simulink model "FlameAnalysis"  (R2015b)
settings: Solver=ode45  SolverMode=SingleTasking  StartTime=0.0  StopTime=1000  RelTol=1e-3
PreLoadFcn:
  | fprintf('loading now...\n')
PostLoadFcn:
  | model_name = gcs;
  | video_player_name=[model_name, '/From Multimedia File'];
  | video_path=get_param(video_player_name,'inputFileName');
  | model_path= get_param(model_name,'filename');
  | i=findstr('\',model_path);
  | 
  | if(~exist(video_path))
  |      video_path2=[model_path(1:i(end))  video_path(findstr('Video',video_path):end)];
  | 
  |      if(exist(video_path2))
  |           set_param(video_player_name,'inputFileName',video_path2);
  |      else
  |           j=findstr('\',video_path);
  |           video_path2=[model_path(1:i(end))  'Videos\' video_path(j(end)+1:end)];
  |           if(exist(video_path2))
  |                set_param(video_player_name,'inputFileName',video_path2);
  |           else
  |                avifiles=dir('videos\*.avi')
  |                set_param(video_player_name,'inputFileName',[model_path(1:i(end))  'Videos\'   avifiles(1).name]);
  |           end
  | 
  |      end
  | end
InitFcn:
  | clc
  | clear
  | global  t position wide dz_dt d2z_dt2 d3z_dt3 Af As dA_dt filePath Su_ Su alfa Karlovitz threshold model_name bords tWalls sheet model_path simulating numPointsAnalysis
  | simulating=true;
  | model_name = gcs;
  | model_path = [model_name, '/Edit Parameters'];
  | tbf = str2num(get_param(model_path,'tbf'));
  | ppcm= str2num(get_param(model_path,'ppcm'));
  | p2e= str2num(get_param(model_path,'p2e'));
  | 
  | nframes0= str2num(get_param(model_path,'nframes0'));
  | alfa= str2num(get_param(model_path,'alfa'));
  | fff= str2num(get_param(model_path,'fff'));
  | 
  | if((size(fff,2)~=1) & (size(fff,2)~=2))
  |     error('The flame front fraction must be scalar or 1x2-array');
  | end
  | order=str2num(get_param(model_path,'order'));
  | numberOfPoints=str2num(get_param(model_path,'numberOfPoints'));
  | orderAnalysis=str2num(get_param(model_path,'orderAnalysis'));
  | numPointsAnalysis=str2num(get_param(model_path,'numPointsAnalysis'));
  | uselog=str2num(get_param(model_path,'uselog'));
  | 
  | 
  | save2xls= strcmp('on',get_param(model_path,'save2xls'));
  | saveVideo= strcmp('on',get_param(model_path,'saveVideo'));
  | cfs= strcmp('on',get_param(model_path,'cfs'));
  | c3dv= strcmp('on',get_param(model_path,'c3dv'));
  | 
  | 
  | if(strcmp(get_param(model_path,'bge'),'Temporal Median Estimator'))
  |      bge=1;
  | elseif (strcmp(get_param(model_path,'bge'),'Temporal Median'))
  |     bge=2;
  |     bkgnd{1}=[gcs '/Background Estimator/Decomposing Red Movement/BG1/Temporal Median/Temporal Median'];
  |     bkgnd{2}=[gcs '/Background Estimator/Decomposing Green Movement/BG1/Temporal Median/Temporal Median'];
  |     bkgnd{3}=[gcs '/Background Estimator/Decomposing Blue Movement/BG1/Temporal Median/Temporal Median'];
  | 
  |     nframes0=max(nframes0,1);
  |     set_param([gcs '/Edit Parameters/'],'nframes0',num2str(nframes0));
  |     for i=1:3
  |         set_param(bkgnd{i}, 'tw', num2str(nframes0));
  |     end
  | else
  |     bge=3;
  | end
  | 
  | 
  | 
  | switch(get_param(model_path,'aprox_type'))
  |      case 'Profile'
  |            aprox_type=1;
  |            sheet='Profile';
  |      case 'Paraboloid (moving base)'
  |            aprox_type=2;
  |            sheet='Paraboloid';
  |      case 'Paraboloid(fixed base)'
  |            aprox_type=3;
  |            sheet='ParaboloidFB';
  |      case 'Spheroid'
  |            aprox_type=4;
  |            sheet='Spheroid';
  |      case 'Profile Spheroid'
  |            aprox_type=5;
  |            sheet='Profile Spheroid';
  | end
  | 
  | 
  | video_player_name=[model_name, '/From Multimedia File'];
  | video_path=get_param(video_player_name,'inputFileName');
  | video_name=getVideoNameFromPath(video_path);
  | hVideoSrc = vision.VideoFileReader(video_path, ...
  |                    'ImageColorSpace','Intensity');
  | firstFrame=step(hVideoSrc);
  | clear hVideoSrc;
  | [m n]=size(firstFrame);
  | 
  | 
  | set_param([model_name '/Display Results/Save Video/modified video/'],'outputFilename',['Videos Matlab/' video_name '_' get_param(model_path,'aprox_type') '_Matlab.avi']);
StopFcn:
  | global editing  simulating
  | simulating = true;
  | try
  |       closeFunction
  | catch err
  |       simulating=false;
  |       err
  | end
  |   simulating=false;
model workspace (MATLAB code in the model file):
  | line_row =  22;
values from neighbouring files (symbols this model uses):
  m = size(BW,1)    [flameFront.m]    (also in putCircles.m = (y(i+1)-y(i))./(x(i+1)-x(i)))
  n = n(n==size(num,2)/4)    [averageOfVideos.m]    (also in countFramesOfVideo.m = 1; putCircles.m = length(y))
  vector = cast([row, col],'double')    [flameFront.m]
undefined symbols (not defined in the file or in its folder): strel
libraries: simulink x27, visionstatistics x14, visionconversions x9, visiontextngfix x9, visionmorphops x7, dspvision x4, visionsinks x2, visiongeotforms x1
(part 1 of 3)
CloseFcn:
  | fprintf('closing now...\n')
settings Model: NumberOfSteps=10  ExtModeAutoUpdateStatusClock=off  Creator=don  LastModifiedBy=nicku
settings DataIOCC: SaveFormat=Array
settings OptimizationCC: BlockReduction=off  BooleanDataType=off
settings DebuggingCC: SaveWithParameterizedLinksMsg=none  UnderspecifiedInitializationDetection=Classic  MergeDetectMultiDrivingBlocksExec=none
settings HardwareCC: ProdBitPerPointer=32  ProdLargestAtomicFloat=None  ProdIntDivRoundTo=Undefined  ProdEndianess=Unspecified  ProdWordSize=32  ProdHWDeviceType=32-bit Generic  TargetUnknown=on
settings GRTTargetCC: GeneratePreprocessorConditionals=Disable all
settings ConfigComp: CovModelRefEnable=Off  CovSFcnEnable=off

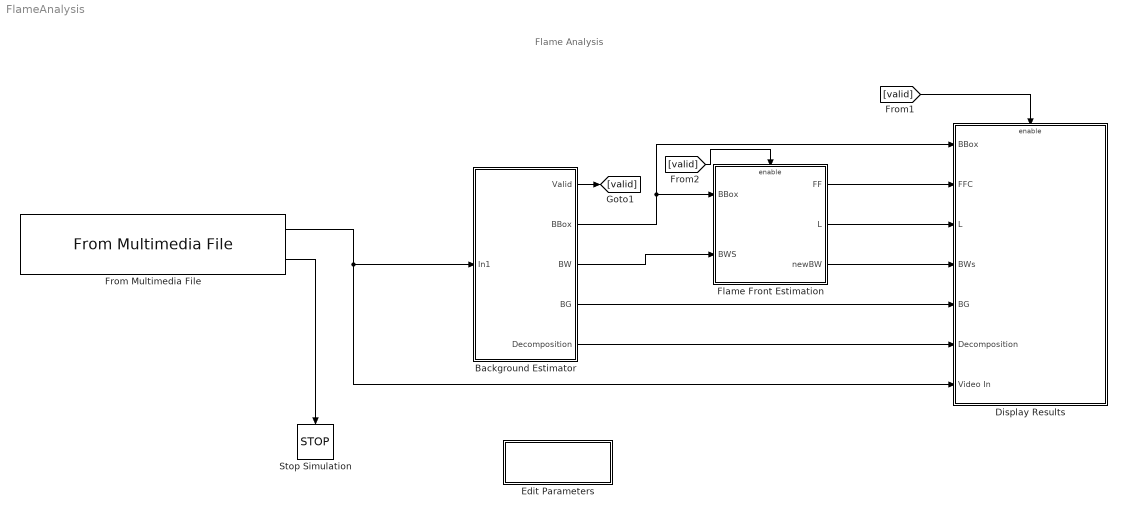
== system FlameAnalysis ==
  note: Flame Analysis
  Background Estimator : Subsystem
  Display Results : Subsystem
  Edit Parameters : Subsystem  mask(Edit Parameters){saveVideo=on, save2xls=on, cfs=on, c3dv=off, bge=Temporal Median, nframes0=52, fff=[0.95        0.93], tbf=200, ppcm=(781 -84)/85, p2e=88, alfa=951.18/293.15, numberOfPoints=10, order=3, aprox_type=Profile Spheroid, splinesmoothing=Spline Smoothing (matlab), numPointsAnalysis=[0.95        0.98       0.001], orderAnalysis=[3  3], uselog=[2  2  1]}
      mask prompts: saveVideo "Save Video"; save2xls "Save Data to excel"; cfs "Calculate Flame Surface"; c3dv "Create 3D video"; bge "Background Estimator"; nframes0 "Number of initial frames"; fff "Flame Front Fraction (0-1)"; tbf "Time Between Frames (microsecs)"; ppcm "Pixels per centimeter (cm^ -1)"; p2e "Number of pixels between the bottom and the electrodes"; numberOfPoints "Number of Points for regression of Flame Profile"; order "Order Of  polynomial regresion of flame profile"; aprox_type "Type of aproximation for flame front"; splinesmoothing "Method for ploynomial regression"; numPointsAnalysis "Smoothing Parameter"; orderAnalysis "Order of polynomia for data regresion  for area and position derivatives"; uselog "Use regression logaritms"
      mask init:
      | % global editing smoothing
      | % model_path=[gcs '/Edit Parameters'];
      | % smoothing=strcmp(get_param(model_path,'splinesmoothing'),'Spline Smoothing (matlab)');
      | % if ~editing
      | %     
      | % 
      | % a=getSimulinkBlockHandle(model_path,true);
      | % masknames=get(a, 'masknames'); 
      | % maskprompts=get(a, 'maskprompts');
      | % maskvisibilities=get(a, 'maskvisibilities');
      | % 
      | % inp=cellfun(@(x)strcmp(x,'numPointsAnalysis'),masknames);
      | % ioa=cellfun(@(x)strcmp(x,'orderAnalysis'),masknames);
      | % 
      | % 
      | % if strcmp(get_param(model_path,'splinesmoothing'),'Spline Smoothing (matlab)')
      | %     maskprompts{inp}='Smoothing Parameter';
      | %     maskvisibilities{ioa}='off';
      | %     set_param(model_path,'numPointsAnalysis',['[' num2str(10.^(log10(str2num(get_param(model_path,'numPointsAnalysis')))+4)) ']']);
      | % else
      | %     maskprompts{inp}='Number of Points for regression of Flame Profile';
      | %     maskvisibilities{ioa}='on';
      | %     set_param(model_path,'numPointsAnalysis',['[' num2str(round(10.^(log10(str2num(get_param(model_path,'numPointsAnalysis')))-4))) ']']);
      | % end
      | % 
      | % set(a,'maskprompts',maskprompts);
      | % set(a,'maskvisibilities',maskvisibilities);
      | % 
      | % end
      settings: RTWMemSecFuncInitTerm=Default  RTWMemSecFuncExecute=Default  RTWMemSecDataConstants=Default  RTWMemSecDataInternal=Default  RTWMemSecDataParameters=Default
      mask TypeOptions bge: Temporal Median Estimator | Temporal Median | Motion Based Background Estimator
      mask TypeOptions aprox_type: Profile | Paraboloid (moving base) | Paraboloid(fixed base) | Spheroid | Profile Spheroid
      mask TypeOptions splinesmoothing: Spline Smoothing (matlab) | multipolyfit  (nicolas' sad try to do what matlab already does)
      mask Callback splinesmoothing:
      | % global editing smoothing
      | % model_path=[gcs '/Edit Parameters'];
      | % if ~editing & strcmp(get_param(model_path,'splinesmoothing'),'Spline Smoothing (matlab)')~=smoothing
      | %     model_path=[gcs '/Edit Parameters'];
      | %
      | % a=getSimulinkBlockHandle(model_path,true);
      | % masknames=get(a, 'masknames');
      | % maskprompts=get(a, 'maskprompts');
      | % maskvisibilities=get(a, 'maskvisibilities');
      | %
      | % inp=cellfun(@(x)strcmp(x,'numPointsAnalysis'),masknames);
      | % ioa=cellfun(@(x)strcmp(x,'orderAnalysis'),masknames);
      | %
      | %
      | % if strcmp(get_param(model_path,'splinesmoothing'),'Spline Smoothing (matlab)')
      | %     maskprompts{inp}='Smoothing Parameter';
      | %     maskvisibilities{ioa}='off';
      | %     set_param(model_path,'numPointsAnalysis',['[' num2str(10.^(log10(str2num(get_param(model_path,'numPointsAnalysis')))-4)) ']']);
      | % else
      | %     maskprompts{inp}='Number of Points for regression of Flame Profile';
      | %     maskvisibilities{ioa}='on';
      | %     set_param(model_path,'numPointsAnalysis',['[' num2str(round(10.^(log10(str2num(get_param(model_path,'numPointsAnalysis')))+4))) ']']);
      | % end
      | %
      | % set(a,'maskprompts',maskprompts);
      | % set(a,'maskvisibilities',maskvisibilities);
      | %
      | % end
      | % smoothing= strcmp(get_param(model_path,'splinesmoothing'),'Spline Smoothing (matlab)');
      mask Display: disp('Edit\nParameters')
  Flame Front Estimation : Subsystem
  From Multimedia File : dspvision/From Multimedia File  inputFilename=D:\Documents\LRGP\GitHub\Flame Detection\Videos\Amidon_319mg_Methane_8.47%_tv120ms_1000mJ_2VD.avi  loop=on  numPlays=2  outputStreams=Video only  videoDataType=single  audioDataType=int16  inheritSampleTime=on  userDefinedSampleTime=1/40  noAudioOutput=off  isIntensityVideo=off  fourcc=RGB  colorVideoFormat=One multidimensional signal  outputEOF=on  dataOrg=Column-major  audioFrameSize=1024  computeAudioFrameSize=off  outSamplingMode=Frame based
  Stop Simulation : Stop
  wires:
  [valid] -> Flame Front Estimation/Enable
  Flame Front Estimation/1(FF) -> Display Results/2(FFC)
  From Multimedia File/2 -> Stop Simulation/1
  Flame Front Estimation/2(L) -> Display Results/3(L)
  [valid] -> Display Results/Enable
  Flame Front Estimation/3(newBW) -> Display Results/4(BWs)
  Background Estimator/2(BBox) -> Display Results/1(BBox), Flame Front Estimation/1(BBox)
  Background Estimator/1(Valid) -> [valid]
  Background Estimator/3(BW) -> Flame Front Estimation/2(BWS)
  Background Estimator/4(BG) -> Display Results/5(BG)
  From Multimedia File/1 -> Display Results/7(Video In), Background Estimator/1(In1)
  Background Estimator/5(Decomposition) -> Display Results/6(Decomposition)

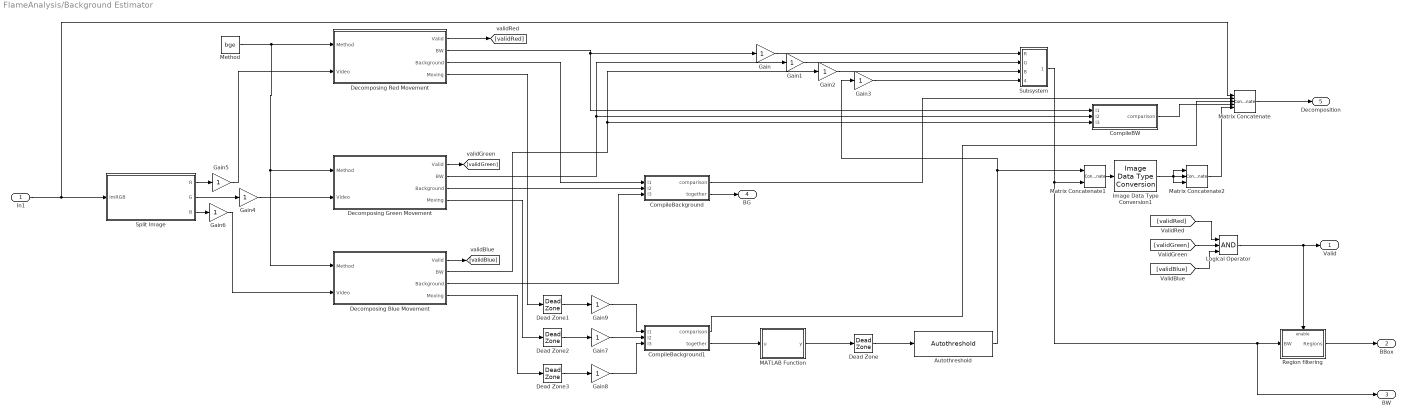
== system FlameAnalysis/Background Estimator ==
  In1 : Inport
  Autothreshold : visionconversions/Autothreshold  operator=>  threshOut=off  effMetricOut=off  userDefinedRange=off  umin=0  umax=255  outOfRngOpt=Warn and saturate  scaleThreshold=off  scaleFactor=0.011  P1Mode=Specify word length  P1WordLength=32  P1FracLength=30  P2Mode=Specify word length  P2WordLength=32  P2FracLength=22  P3Mode=Specify word length  P3WordLength=32  P3FracLength=14  P4Mode=Binary point scaling  P4WordLength=32  P4FracLength=15  Q1Mode=Specify word length  Q1WordLength=32  Q1FracLength=16  EMMode=Specify word length  EMWordLength=16  EMFracLength=14  roundingMode=Floor  overflowMode=off
  CompileBW : MATLAB Function  TreatAsAtomicUnit=on
  CompileBackground : MATLAB Function  TreatAsAtomicUnit=on
  CompileBackground1 : MATLAB Function  TreatAsAtomicUnit=on
  Dead Zone{,1..3} (4 alike) : DeadZone  LowerValue=0  UpperValue=0  SaturateOnIntegerOverflow=on
  Decomposing Blue Movement : Subsystem
  Decomposing Green Movement : Subsystem
  Decomposing Red Movement : Subsystem
  Gain{,1..9} (10 alike) : Gain
  Image Data Type Conversion1 : visionconversions/Image Data Type Conversion  outDT=single  isSigned=on  wordLen=16  numFracBits=0
  Logical Operator : Logic  Inputs=3  AllPortsSameDT=off  OutDataTypeStr=boolean
  MATLAB Function : MATLAB Function  TreatAsAtomicUnit=on
  Matrix Concatenate : Concatenate  NumInputs=5  Mode=Multidimensional array
  Matrix Concatenate1 : Concatenate  Mode=Multidimensional array
  Matrix Concatenate2 : Concatenate  NumInputs=3  Mode=Multidimensional array  ConcatenateDimension=3
  Method : Constant  Value=bge  OutDataTypeStr=single
  Region filtering : Subsystem
      settings: RTWMemSecFuncInitTerm=Default  RTWMemSecFuncExecute=Default  RTWMemSecDataConstants=Default  RTWMemSecDataInternal=Default  RTWMemSecDataParameters=Default
  Split Image : MATLAB Function  TreatAsAtomicUnit=on
  Subsystem : Subsystem
  Valid : Outport
  BBox : Outport  Port=2
  BW : Outport  Port=3
  BG : Outport  Port=4
  Decomposition : Outport  Port=5
  wires:
  Logical Operator/1 -> Valid/1, Region filtering/Enable
  Region filtering/1(Regions) -> BBox/1
  Subsystem/1(BW) -> Matrix Concatenate1/2, BW/1, Region filtering/1(BW)
  CompileBackground/2(together) -> BG/1
  Method/1 -> Decomposing Blue Movement/1(Method), Decomposing Green Movement/1(Method), Decomposing Red Movement/1(Method)
  Decomposing Red Movement/2(BW) -> CompileBW/1(I1), Gain/1
  Decomposing Red Movement/3(Background) -> CompileBackground/1(I1)
  Decomposing Red Movement/1(Valid) -> [validRed]
  Decomposing Green Movement/1(Valid) -> [validGreen]
  Decomposing Blue Movement/1(Valid) -> [validBlue]
  [validRed] -> Logical Operator/1
  [validGreen] -> Logical Operator/2
  [validBlue] -> Logical Operator/3
  Decomposing Green Movement/3(Background) -> CompileBackground/2(I2)
  Decomposing Blue Movement/3(Background) -> CompileBackground/3(I3)
  Decomposing Green Movement/2(BW) -> Gain1/1, CompileBW/2(I2)
  Decomposing Blue Movement/2(BW) -> Gain2/1, CompileBW/3(I3)
  Matrix Concatenate/1 -> Decomposition/1
  CompileBackground1/2(together) -> MATLAB Function/1(u)
  CompileBackground/1(comparison) -> Matrix Concatenate/2
  CompileBackground1/1(comparison) -> Matrix Concatenate/3
  CompileBW/1(comparison) -> Matrix Concatenate/4
  Matrix Concatenate2/1 -> Matrix Concatenate/5
  Gain/1 -> Subsystem/1(R)
  Gain1/1 -> Subsystem/2(G)
  Gain2/1 -> Subsystem/3(B)
  Gain3/1 -> Subsystem/4(RGB)
  Autothreshold/1 -> Gain3/1, Matrix Concatenate1/1
  Matrix Concatenate1/1 -> Image Data Type Conversion1/1
  Image Data Type Conversion1/1 -> Matrix Concatenate2/1, Matrix Concatenate2/3, Matrix Concatenate2/2
  Split Image/1(R) -> Gain5/1
  Split Image/2(G) -> Gain4/1
  Split Image/3(B) -> Gain6/1
  Decomposing Green Movement/4(Moving) -> Dead Zone2/1
  Decomposing Blue Movement/4(Moving) -> Dead Zone3/1
  Decomposing Red Movement/4(Moving) -> Dead Zone1/1
  In1/1 -> Matrix Concatenate/1, Split Image/1(imRGB)
  Gain4/1 -> Decomposing Green Movement/2(Video)
  Gain5/1 -> Decomposing Red Movement/2(Video)
  Gain6/1 -> Decomposing Blue Movement/2(Video)
  Dead Zone/1 -> Autothreshold/1
  MATLAB Function/1(y) -> Dead Zone/1
  Dead Zone1/1 -> Gain9/1
  Dead Zone2/1 -> Gain7/1
  Dead Zone3/1 -> Gain8/1
  Gain7/1 -> CompileBackground1/2(I2)
  Gain8/1 -> CompileBackground1/3(I3)
  Gain9/1 -> CompileBackground1/1(I1)

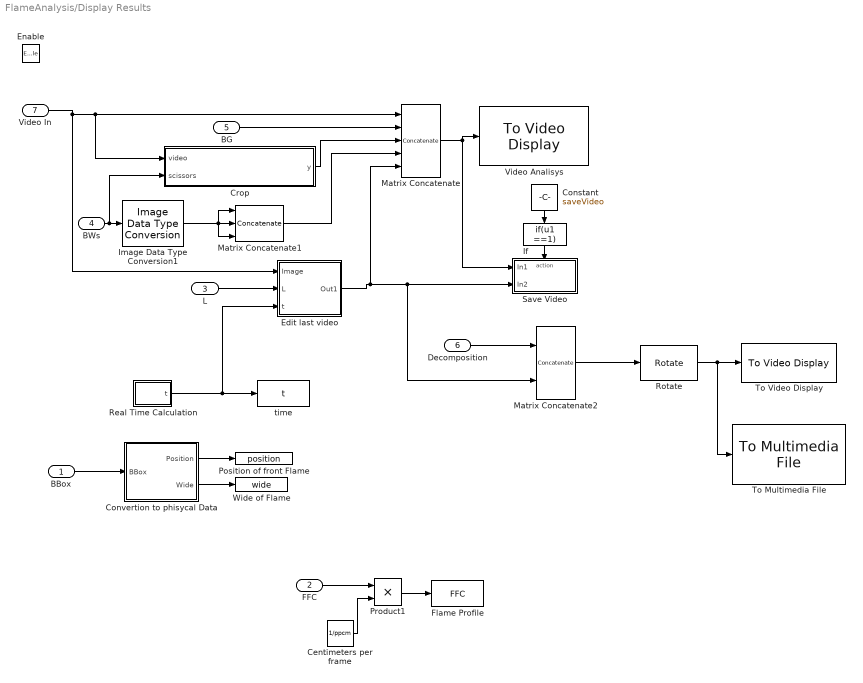
== system FlameAnalysis/Display Results ==
  BBox : Inport
  FFC : Inport  Port=2
  L : Inport  Port=3
  BWs : Inport  Port=4
  BG : Inport  Port=5
  Decomposition : Inport  Port=6
  Video In : Inport  Port=7
  Enable : EnablePort  PropagateVarSize=During execution
  Centimeters per frame : Constant  Value=1/ppcm
  Constant : Constant  Value=saveVideo
  Convertion to phisycal Data : Subsystem
  Crop : MATLAB Function  TreatAsAtomicUnit=on
  Edit last video : Subsystem
  Flame Profile : ToWorkspace  VariableName=FFC  SaveFormat=Structure With Time  SampleTime=-1
  If : If  IfExpression=u1 ==1  ShowElse=off
  Image Data Type Conversion1 : visionconversions/Image Data Type Conversion  outDT=single  isSigned=on  wordLen=16  numFracBits=0
  Matrix Concatenate : Concatenate  NumInputs=5  Mode=Multidimensional array
  Matrix Concatenate1 : Concatenate  NumInputs=3  Mode=Multidimensional array  ConcatenateDimension=3
  Matrix Concatenate2 : Concatenate  Mode=Multidimensional array
  Position of front Flame : ToWorkspace  VariableName=position  SampleTime=-1
  Product1 : Product  RndMeth=Zero
  Real Time Calculation : Subsystem
  Rotate : visiongeotforms/Rotate  outSizeR=Expanded to fit rotated input image  src_angle=Specify via dialog  unit_angle=Degrees  angle=pi/2  maxAngle=pi  dispImage=Center  method=Table lookup  fillVal=0  interpMethod=Bilinear  prodOutputMode=Binary point scaling  prodOutputWordLength=32  prodOutputFracLength=10  roundingMode=Nearest  overflowMode=on
  Save Video : Subsystem  TreatAsAtomicUnit=on
  To Multimedia File : dspvision/To Multimedia File  outputFilename=Videos Matlab\decomposition.avi  streamSelection=Video only  videoCompressor=None (uncompressed)  audioCompressor=None (uncompressed)  imagePorts=One multidimensional signal  fileType=AVI  audioDatatype=Determine from input data type  fourcc=RGB  videoQuality=75  mj2000CompFactor=10
  To Video Display : visionsinks/To Video Display  windowSizeMode=True size (1:1)  openAtMdlStart=on  fullScreen=off  videoWindowX=-1920  videoWindowY=-104  saveWindowSize=off  videoWindowWidth=1920  videoWindowHeight=1017  inputColorFormat=RGB  inputType=Obsolete  imagePorts=One multidimensional signal  OutputDevice=On-screen video monitor  dataOrg=Column-major  isWindowOpen=on
  Video Analisys : visionsinks/To Video Display  windowSizeMode=True size (1:1)  openAtMdlStart=on  fullScreen=off  videoWindowX=0  videoWindowY=23  saveWindowSize=off  videoWindowWidth=1366  videoWindowHeight=705  inputColorFormat=RGB  inputType=Obsolete  imagePorts=One multidimensional signal  OutputDevice=On-screen video monitor  dataOrg=Column-major  isWindowOpen=on
  Wide of Flame : ToWorkspace  VariableName=wide  SampleTime=-1
  time : ToWorkspace  VariableName=t  SampleTime=-1
  wires:
  BWs/1 -> Crop/2(scissors), Image Data Type Conversion1/1
  Matrix Concatenate/1 -> Save Video/1(In1), Video Analisys/1
  Video In/1 -> Edit last video/1(Image), Crop/1(video), Matrix Concatenate/1
  BBox/1 -> Convertion to phisycal Data/1(BBox)
  Convertion to phisycal Data/1(Position) -> Position of front Flame/1
  Convertion to phisycal Data/2(Wide) -> Wide of Flame/1
  Constant/1 -> If/1
  If/1 -> Save Video/Action
  Real Time Calculation/1(t) -> time/1, Edit last video/3(t)
  FFC/1 -> Product1/1
  Centimeters per frame/1 -> Product1/2
  Product1/1 -> Flame Profile/1
  Edit last video/1(Out1) -> Matrix Concatenate/5, Matrix Concatenate2/2, Save Video/2(In2)
  L/1 -> Edit last video/2(L)
  Image Data Type Conversion1/1 -> Matrix Concatenate1/1, Matrix Concatenate1/3, Matrix Concatenate1/2
  BG/1 -> Matrix Concatenate/2
  Matrix Concatenate1/1 -> Matrix Concatenate/4
  Crop/1(y) -> Matrix Concatenate/3
  Decomposition/1 -> Matrix Concatenate2/1
  Rotate/1 -> To Multimedia File/1, To Video Display/1
  Matrix Concatenate2/1 -> Rotate/1

== system FlameAnalysis/Edit Parameters ==

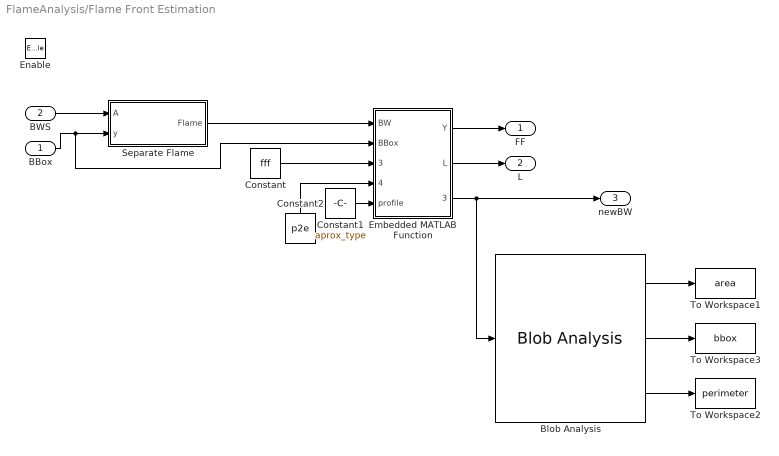
== system FlameAnalysis/Flame Front Estimation ==
  BBox : Inport
  BWS : Inport  Port=2
  Enable : EnablePort  PropagateVarSize=During execution
  Blob Analysis : visionstatistics/Blob Analysis  Tag=vipblks_row_conv  area=on  centroid=off  bBox=on  majorAxis=off  minorAxis=off  angle=off  eccentricity=off  equivDiameterSq=off  extent=off  perimeter=on  maxBlobs=1  warnIfNumBlobsExceeded=on  isCount=off  useMinArea=off  minArea=5*5  useMaxArea=off  maxArea=intmax('uint32')  excludeBorderBlob=off  outDT=double  isOutVarDim=off  isFill=on  fillValues=-1  conn=8  isLabel=off  outputMode=Binary point scaling  outputWordLength=32  outputFracLength=16  firstCoeffMode=Binary point scaling  firstCoeffWordLength=16  firstCoeffFracLength=14  secondCoeffMode=Binary point scaling  secondCoeffWordLength=32  secondCoeffFracLength=16  accumMode=Binary point scaling  accumWordLength=32  accumFracLength=0  prodOutputMode=Binary point scaling  prodOutputWordLength=32  prodOutputFracLength=16  roundingMode=Floor  overflowMode=off
  Constant : Constant  Value=fff  VectorParams1D=off
  Constant1 : Constant  Value=aprox_type  VectorParams1D=off
  Constant2 : Constant  Value=p2e  VectorParams1D=off
  Embedded MATLAB Function : MATLAB Function  TreatAsAtomicUnit=on
  Separate Flame : MATLAB Function  TreatAsAtomicUnit=on
  To Workspace1 : ToWorkspace  VariableName=area  SampleTime=-1
  To Workspace2 : ToWorkspace  VariableName=perimeter  SampleTime=-1
  To Workspace3 : ToWorkspace  VariableName=bbox  SampleTime=-1
  FF : Outport
  L : Outport  Port=2
  newBW : Outport  Port=3
  wires:
  BWS/1 -> Separate Flame/1(A)
  BBox/1 -> Separate Flame/2(y), Embedded MATLAB Function/2(BBox)
  Separate Flame/1(Flame) -> Embedded MATLAB Function/1(BW)
  Constant/1 -> Embedded MATLAB Function/3(fraction)
  Constant1/1 -> Embedded MATLAB Function/5(profile)
  Embedded MATLAB Function/1(Y) -> FF/1
  Embedded MATLAB Function/2(L) -> L/1
  Constant2/1 -> Embedded MATLAB Function/4(y_electrodes)
  Embedded MATLAB Function/3(newBW) -> Blob Analysis/1, newBW/1
  Blob Analysis/1 -> To Workspace1/1
  Blob Analysis/3 -> To Workspace2/1
  Blob Analysis/2 -> To Workspace3/1

== system FlameAnalysis/Background Estimator/Decomposing Blue Movement ==
  Method : Inport
  Video : Inport  Port=2
  BG1 : Subsystem
  Movement Tracker : Subsystem
  Valid : Outport
  BW : Outport  Port=2
  Background : Outport  Port=3
  Moving : Outport  Port=4
  wires:
  Video/1 -> BG1/2(Video), Movement Tracker/2(Video In 1)
  Method/1 -> BG1/1(Constant)
  BG1/2(Background) -> Background/1, Movement Tracker/1(Background 1)
  Movement Tracker/2(BW) -> BW/1
  BG1/1(Valid) -> Movement Tracker/Enable, Valid/1
  Movement Tracker/1(Moving) -> Moving/1

== system FlameAnalysis/Background Estimator/Decomposing Green Movement ==
  Method : Inport
  Video : Inport  Port=2
  BG1 : Subsystem
  Movement Tracker : Subsystem
  Valid : Outport
  BW : Outport  Port=2
  Background : Outport  Port=3
  Moving : Outport  Port=4
  wires:
  Video/1 -> BG1/2(Video), Movement Tracker/2(Video In 1)
  Movement Tracker/1(Moving) -> Moving/1
  Method/1 -> BG1/1(Constant)
  BG1/2(Background) -> Background/1, Movement Tracker/1(Background 1)
  Movement Tracker/2(BW) -> BW/1
  BG1/1(Valid) -> Movement Tracker/Enable, Valid/1

== system FlameAnalysis/Background Estimator/Decomposing Red Movement ==
  Method : Inport
  Video : Inport  Port=2
  BG1 : Subsystem
  Movement Tracker : Subsystem
  Valid : Outport
  BW : Outport  Port=2
  Background : Outport  Port=3
  Moving : Outport  Port=4
  wires:
  Video/1 -> BG1/2(Video), Movement Tracker/2(Video In 1)
  Movement Tracker/1(Moving) -> Moving/1
  Method/1 -> BG1/1(Constant)
  BG1/2(Background) -> Background/1, Movement Tracker/1(Background 1)
  Movement Tracker/2(BW) -> BW/1
  BG1/1(Valid) -> Movement Tracker/Enable, Valid/1

== system FlameAnalysis/Background Estimator/Region filtering ==
  BW : Inport
  Enable : EnablePort  PropagateVarSize=During execution
  Blob Analysis : visionstatistics/Blob Analysis  Tag=vipblks_row_conv  area=on  centroid=off  bBox=on  majorAxis=off  minorAxis=off  angle=off  eccentricity=off  equivDiameterSq=off  extent=off  perimeter=off  maxBlobs=1000  warnIfNumBlobsExceeded=on  isCount=off  useMinArea=off  minArea=5*5  useMaxArea=on  maxArea=int32(0.9*m*n)  excludeBorderBlob=off  outDT=double  isOutVarDim=off  isFill=on  fillValues=0  conn=8  isLabel=off  outputMode=Binary point scaling  outputWordLength=32  outputFracLength=16  firstCoeffMode=Binary point scaling  firstCoeffWordLength=16  firstCoeffFracLength=14  secondCoeffMode=Binary point scaling  secondCoeffWordLength=32  secondCoeffFracLength=16  accumMode=Binary point scaling  accumWordLength=32  accumFracLength=0  prodOutputMode=Binary point scaling  prodOutputWordLength=32  prodOutputFracLength=16  roundingMode=Floor  overflowMode=off
  blobDepurator : MATLAB Function  TreatAsAtomicUnit=on
  Regions : Outport
  wires:
  BW/1 -> Blob Analysis/1
  Blob Analysis/2 -> blobDepurator/2(blobs)
  Blob Analysis/1 -> blobDepurator/1(areas)
  blobDepurator/1(Y) -> Regions/1

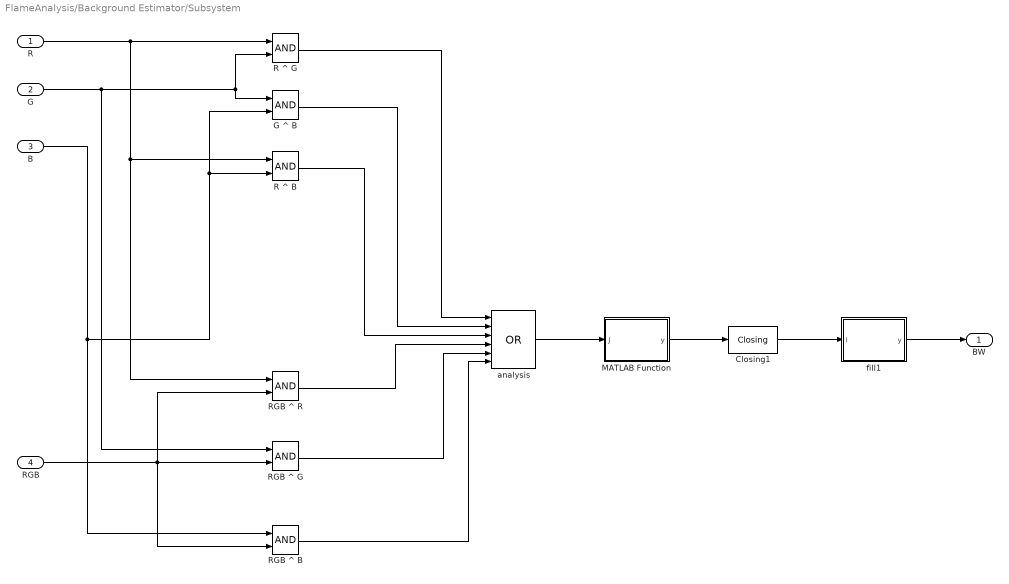
== system FlameAnalysis/Background Estimator/Subsystem ==
  R : Inport
  G : Inport  Port=2
  B : Inport  Port=3
  RGB : Inport  Port=4
  Closing1 : visionmorphops/Closing  nhoodsrc=Specify via dialog  strel=strel('disk',3)
  G ^ B : Logic  AllPortsSameDT=off  OutDataTypeStr=boolean
  MATLAB Function : MATLAB Function  TreatAsAtomicUnit=on
  R ^ B : Logic  AllPortsSameDT=off  OutDataTypeStr=boolean
  R ^ G : Logic  AllPortsSameDT=off  OutDataTypeStr=boolean
  RGB ^ B : Logic  AllPortsSameDT=off  OutDataTypeStr=boolean
  RGB ^ G : Logic  AllPortsSameDT=off  OutDataTypeStr=boolean
  RGB ^ R : Logic  AllPortsSameDT=off  OutDataTypeStr=boolean
  analysis : Logic  Operator=OR  Inputs=6  AllPortsSameDT=off  OutDataTypeStr=boolean
  fill1 : MATLAB Function  TreatAsAtomicUnit=on
  BW : Outport
  wires:
  R/1 -> RGB ^ R/1, R ^ B/1, R ^ G/1
  G/1 -> RGB ^ G/1, G ^ B/1, R ^ G/2
  B/1 -> RGB ^ B/1, R ^ B/2, G ^ B/2
  R ^ G/1 -> analysis/1
  G ^ B/1 -> analysis/2
  R ^ B/1 -> analysis/3
  analysis/1 -> MATLAB Function/1(J)
  RGB/1 -> RGB ^ B/2, RGB ^ G/2, RGB ^ R/2
  RGB ^ R/1 -> analysis/4
  RGB ^ G/1 -> analysis/5
  RGB ^ B/1 -> analysis/6
  MATLAB Function/1(y) -> Closing1/1
  fill1/1(y) -> BW/1
  Closing1/1 -> fill1/1(I)

== system FlameAnalysis/Display Results/Convertion to phisycal Data ==
  BBox : Inport
  Array To Scalar : MATLAB Function  TreatAsAtomicUnit=on
  Centimeters per frame : Constant  Value=1/ppcm
  pixels to electrodes : Constant  Value=p2e
  Position : Outport
  Wide : Outport  Port=2
  wires:
  Array To Scalar/1(position) -> Position/1
  BBox/1 -> Array To Scalar/1(u)
  pixels to electrodes/1 -> Array To Scalar/3(p2e)
  Centimeters per frame/1 -> Array To Scalar/2(cmpf)
  Array To Scalar/2(wide) -> Wide/1

== system FlameAnalysis/Display Results/Edit last video ==
  Image : Inport
  L : Inport  Port=2
  t : Inport  Port=3
  Constant : Constant  Value=int32([n/2-35 m-20 80 30])
  Draw Shapes : visiontextngfix/Draw Shapes  shape=Rectangles  fill=on  lineWidth=1  fillClrSource=Specify via dialog  display=Black  intensity=200  color=[255 0 0]  opacity=1  viewport=Entire image  antialiasing=off  inType=Obsolete  imagePorts=One multidimensional signal  prodOutputMode=Binary point scaling  prodOutputWordLength=32  prodOutputFracLength=14  memoryMode=Specify word length  memoryWordLength=16  memoryFracLength=14  roundingMode=Floor  overflowMode=off
  Draw Shapes1 : visiontextngfix/Draw Shapes  shape=Lines  fill=off  lineWidth=1  fillClrSource=Specify via dialog  display=User-specified value  intensity=200  color=[ 0 0 0]  opacity=0.6  viewport=Entire image  antialiasing=off  inType=Obsolete  imagePorts=One multidimensional signal  prodOutputMode=Binary point scaling  prodOutputWordLength=32  prodOutputFracLength=14  memoryMode=Specify word length  memoryWordLength=16  memoryFracLength=14  roundingMode=Floor  overflowMode=off
  Insert Text : visiontextngfix/Insert Text  inputType=Obsolete  theText=['%6.2f ms']  getTextLocFrom=Specify via dialog  textLoc=int32([n/2-30 m-15])  getTextColorFrom=Specify via dialog  textColor=[1 1 1]  getTextIntensityFrom=Specify via dialog  textIntensity=0  getTextOpacityFrom=Specify via dialog  textOpacity=1.0  dummyVar2=0  dummyVar3=0  dummyVar4=0  imagePorts=One multidimensional signal  isInputTransposed=off  fontFace=LucidaSansRegular  dummyVar1=0  blockFontSize=12  antiAliased=on
  Out1 : Outport
  wires:
  Image/1 -> Draw Shapes1/1
  L/1 -> Draw Shapes1/2
  t/1 -> Insert Text/2
  Insert Text/1 -> Out1/1
  Draw Shapes/1 -> Insert Text/1
  Draw Shapes1/1 -> Draw Shapes/1
  Constant/1 -> Draw Shapes/2

== system FlameAnalysis/Display Results/Real Time Calculation ==
  Constant : Constant  Value=tbf/1000
  Constant1 : Constant
  Frame Counter : Subsystem
  Product : Product  RndMeth=Zero
  Sum : Sum  Inputs=|-+
  t : Outport
  wires:
  Frame Counter/1(" Cnt") -> Sum/2
  Constant/1 -> Product/2
  Constant1/1 -> Sum/1
  Sum/1 -> Product/1
  Product/1 -> t/1

== system FlameAnalysis/Display Results/Save Video ==
  In1 : Inport
  In2 : Inport  Port=2
  Action Port : ActionPort  ActionType=then
  Whole video : dspvision/To Multimedia File  outputFilename=Videos Matlab\results2.avi  streamSelection=Video only  videoCompressor=None (uncompressed)  audioCompressor=None (uncompressed)  imagePorts=One multidimensional signal  fileType=AVI  audioDatatype=Determine from input data type  fourcc=RGB  videoQuality=75  mj2000CompFactor=10
  modified video : dspvision/To Multimedia File  outputFilename=Videos Matlab/Amidon_319mg_Methane_8.47%_tv120ms_1000mJ_2VD_Profile Spheroid_Matlab.avi  streamSelection=Video only  videoCompressor=None (uncompressed)  audioCompressor=None (uncompressed)  imagePorts=One multidimensional signal  fileType=AVI  audioDatatype=Determine from input data type  fourcc=RGB  videoQuality=75  mj2000CompFactor=10
  wires:
  In1/1 -> Whole video/1
  In2/1 -> modified video/1

== system FlameAnalysis/Background Estimator/Decomposing Blue Movement/BG1 ==
  Constant : Inport
  Video : Inport  Port=2
  Compare To Constant : simulink/Logic and Bit Operations/Compare To Constant  relop===  const=1  OutDataTypeStr=boolean  ZeroCross=off
  Compare To Constant1 : simulink/Logic and Bit Operations/Compare To Constant  relop===  const=2  OutDataTypeStr=boolean  ZeroCross=off
  Compare To Constant2 : simulink/Logic and Bit Operations/Compare To Constant  relop===  const=3  OutDataTypeStr=boolean  ZeroCross=off
  Merge : Merge  Inputs=3
  Merge1 : Merge  Inputs=3
  Motion Based Background Estimator : Subsystem
  Temporal Median : Subsystem
  Temporal Median Estimator : Subsystem
  Valid : Outport
  Background : Outport  Port=2
  wires:
  Video/1 -> Motion Based Background Estimator/1(In), Temporal Median/1(In), Temporal Median Estimator/1(In)
  Constant/1 -> Compare To Constant1/1, Compare To Constant2/1, Compare To Constant/1
  Merge1/1 -> Valid/1
  Compare To Constant2/1 -> Motion Based Background Estimator/Enable
  Motion Based Background Estimator/1(BG) -> Merge/3
  Temporal Median Estimator/1(BG) -> Merge/1
  Merge/1 -> Background/1
  Compare To Constant1/1 -> Temporal Median/Enable
  Temporal Median/1(BG) -> Merge/2
  Temporal Median Estimator/2(Valid) -> Merge1/1
  Temporal Median/2(Valid) -> Merge1/2
  Motion Based Background Estimator/2(Valid) -> Merge1/3
  Compare To Constant/1 -> Temporal Median Estimator/Enable

== system FlameAnalysis/Background Estimator/Decomposing Blue Movement/Movement Tracker ==
  Background 1 : Inport
  Video In 1 : Inport  Port=2
  Enable : EnablePort  PropagateVarSize=During execution
  Abs3 : Abs  SaturateOnIntegerOverflow=on
  Autothreshold : visionconversions/Autothreshold  operator=>  threshOut=off  effMetricOut=off  userDefinedRange=off  umin=0  umax=255  outOfRngOpt=Warn and saturate  scaleThreshold=off  scaleFactor=0.011  P1Mode=Specify word length  P1WordLength=32  P1FracLength=30  P2Mode=Specify word length  P2WordLength=32  P2FracLength=22  P3Mode=Specify word length  P3WordLength=32  P3FracLength=14  P4Mode=Binary point scaling  P4WordLength=32  P4FracLength=15  Q1Mode=Specify word length  Q1WordLength=32  Q1FracLength=16  EMMode=Specify word length  EMWordLength=16  EMFracLength=14  roundingMode=Floor  overflowMode=off
  Dead Zone : DeadZone  LowerValue=0  UpperValue=0.05  SaturateOnIntegerOverflow=on
  Gain : Gain
  Sum1 : Sum  Inputs=-+  SaturateOnIntegerOverflow=on  InputSameDT=on  OutDataTypeStr=Inherit: Same as first input
  Moving : Outport
  BW : Outport  Port=2
  wires:
  Video In 1/1 -> Sum1/2
  Sum1/1 -> Abs3/1
  Background 1/1 -> Sum1/1
  Autothreshold/1 -> BW/1
  Dead Zone/1 -> Gain/1
  Abs3/1 -> Dead Zone/1
  Gain/1 -> Moving/1, Autothreshold/1

== system FlameAnalysis/Background Estimator/Decomposing Green Movement/BG1 ==
  Constant : Inport
  Video : Inport  Port=2
  Compare To Constant : simulink/Logic and Bit Operations/Compare To Constant  relop===  const=1  OutDataTypeStr=boolean  ZeroCross=off
  Compare To Constant1 : simulink/Logic and Bit Operations/Compare To Constant  relop===  const=2  OutDataTypeStr=boolean  ZeroCross=off
  Compare To Constant2 : simulink/Logic and Bit Operations/Compare To Constant  relop===  const=3  OutDataTypeStr=boolean  ZeroCross=off
  Merge : Merge  Inputs=3
  Merge1 : Merge  Inputs=3
  Motion Based Background Estimator : Subsystem
  Temporal Median : Subsystem
  Temporal Median Estimator : Subsystem
  Valid : Outport
  Background : Outport  Port=2
  wires:
  Video/1 -> Motion Based Background Estimator/1(In), Temporal Median/1(In), Temporal Median Estimator/1(In)
  Constant/1 -> Compare To Constant1/1, Compare To Constant2/1, Compare To Constant/1
  Merge1/1 -> Valid/1
  Compare To Constant2/1 -> Motion Based Background Estimator/Enable
  Motion Based Background Estimator/1(BG) -> Merge/3
  Temporal Median Estimator/1(BG) -> Merge/1
  Merge/1 -> Background/1
  Compare To Constant1/1 -> Temporal Median/Enable
  Temporal Median/1(BG) -> Merge/2
  Temporal Median Estimator/2(Valid) -> Merge1/1
  Temporal Median/2(Valid) -> Merge1/2
  Motion Based Background Estimator/2(Valid) -> Merge1/3
  Compare To Constant/1 -> Temporal Median Estimator/Enable

== system FlameAnalysis/Background Estimator/Decomposing Green Movement/Movement Tracker ==
  Background 1 : Inport
  Video In 1 : Inport  Port=2
  Enable : EnablePort  PropagateVarSize=During execution
  Abs3 : Abs  SaturateOnIntegerOverflow=on
  Autothreshold : visionconversions/Autothreshold  operator=>  threshOut=off  effMetricOut=off  userDefinedRange=off  umin=0  umax=255  outOfRngOpt=Warn and saturate  scaleThreshold=off  scaleFactor=2  P1Mode=Specify word length  P1WordLength=32  P1FracLength=30  P2Mode=Specify word length  P2WordLength=32  P2FracLength=22  P3Mode=Specify word length  P3WordLength=32  P3FracLength=14  P4Mode=Binary point scaling  P4WordLength=32  P4FracLength=15  Q1Mode=Specify word length  Q1WordLength=32  Q1FracLength=16  EMMode=Specify word length  EMWordLength=16  EMFracLength=14  roundingMode=Floor  overflowMode=off
  Dead Zone : DeadZone  LowerValue=0  UpperValue=0  SaturateOnIntegerOverflow=on
  Gain : Gain
  Sum1 : Sum  Inputs=-+  SaturateOnIntegerOverflow=on  InputSameDT=on  OutDataTypeStr=Inherit: Same as first input
  Moving : Outport
  BW : Outport  Port=2
  wires:
  Video In 1/1 -> Sum1/2
  Sum1/1 -> Abs3/1
  Background 1/1 -> Sum1/1
  Abs3/1 -> Dead Zone/1
  Autothreshold/1 -> BW/1
  Dead Zone/1 -> Gain/1
  Gain/1 -> Autothreshold/1, Moving/1

== system FlameAnalysis/Background Estimator/Decomposing Red Movement/BG1 ==
  Constant : Inport
  Video : Inport  Port=2
  Compare To Constant : simulink/Logic and Bit Operations/Compare To Constant  relop===  const=1  OutDataTypeStr=boolean  ZeroCross=off
  Compare To Constant1 : simulink/Logic and Bit Operations/Compare To Constant  relop===  const=2  OutDataTypeStr=boolean  ZeroCross=off
  Compare To Constant2 : simulink/Logic and Bit Operations/Compare To Constant  relop===  const=3  OutDataTypeStr=boolean  ZeroCross=off
  Merge : Merge  Inputs=3
  Merge1 : Merge  Inputs=3
  Motion Based Background Estimator : Subsystem
  Temporal Median : Subsystem
  Temporal Median Estimator : Subsystem
  Valid : Outport
  Background : Outport  Port=2
  wires:
  Video/1 -> Motion Based Background Estimator/1(In), Temporal Median/1(In), Temporal Median Estimator/1(In)
  Constant/1 -> Compare To Constant1/1, Compare To Constant2/1, Compare To Constant/1
  Merge1/1 -> Valid/1
  Compare To Constant2/1 -> Motion Based Background Estimator/Enable
  Motion Based Background Estimator/1(BG) -> Merge/3
  Temporal Median Estimator/1(BG) -> Merge/1
  Merge/1 -> Background/1
  Compare To Constant1/1 -> Temporal Median/Enable
  Temporal Median/1(BG) -> Merge/2
  Temporal Median Estimator/2(Valid) -> Merge1/1
  Temporal Median/2(Valid) -> Merge1/2
  Motion Based Background Estimator/2(Valid) -> Merge1/3
  Compare To Constant/1 -> Temporal Median Estimator/Enable

== system FlameAnalysis/Background Estimator/Decomposing Red Movement/Movement Tracker ==
  Background 1 : Inport
  Video In 1 : Inport  Port=2
  Enable : EnablePort  PropagateVarSize=During execution
  Abs3 : Abs  SaturateOnIntegerOverflow=on
  Autothreshold : visionconversions/Autothreshold  operator=>  threshOut=off  effMetricOut=off  userDefinedRange=off  umin=0  umax=255  outOfRngOpt=Warn and saturate  scaleThreshold=off  scaleFactor=5  P1Mode=Specify word length  P1WordLength=32  P1FracLength=30  P2Mode=Specify word length  P2WordLength=32  P2FracLength=22  P3Mode=Specify word length  P3WordLength=32  P3FracLength=14  P4Mode=Binary point scaling  P4WordLength=32  P4FracLength=15  Q1Mode=Specify word length  Q1WordLength=32  Q1FracLength=16  EMMode=Specify word length  EMWordLength=16  EMFracLength=14  roundingMode=Floor  overflowMode=off
  Dead Zone : DeadZone  LowerValue=0  UpperValue=0.2  SaturateOnIntegerOverflow=on
  Sum1 : Sum  Inputs=-+  SaturateOnIntegerOverflow=on  InputSameDT=on  OutDataTypeStr=Inherit: Same as first input
  Moving : Outport
  BW : Outport  Port=2
  wires:
  Video In 1/1 -> Sum1/2
  Sum1/1 -> Abs3/1
  Background 1/1 -> Sum1/1
  Autothreshold/1 -> BW/1
  Abs3/1 -> Dead Zone/1
  Dead Zone/1 -> Autothreshold/1, Moving/1

== system FlameAnalysis/Display Results/Real Time Calculation/Frame Counter ==
  Constant : Constant  OutDataTypeStr=int32
  Delay : Delay  DelayLength=1  InitialCondition=0  InputProcessing=Inherited
  Sum : Sum  Inputs=++|  OutDataTypeStr=Inherit: Same as first input
  " Cnt" : Outport
  wires:
  Delay/1 -> Sum/1
  Sum/1 -> " Cnt"/1, Delay/1
  Constant/1 -> Sum/2

== system FlameAnalysis/Background Estimator/Decomposing Blue Movement/BG1/Motion Based Background Estimator ==
  In : Inport
  Enable : EnablePort  PropagateVarSize=During execution
  Motion Based Background Estimator : Subsystem  mask(Motion Based Background Estimation){}
      mask help: The block uses the first few frames of the video stream to estimate the background image. It subtracts the background from each video frame to produce foreground images and only redraws the portion of the background that is revealed by the moving objects.
      mask Display: disp('Motion Based\nBackground\nEstimator')
  Signal Conversion : SignalConversion  ConversionOutput=Contiguous copy
  Signal Conversion1 : SignalConversion  ConversionOutput=Contiguous copy
  BG : Outport
  Valid : Outport  Port=2  InitialOutput=0
  wires:
  Signal Conversion1/1 -> Valid/1
  Signal Conversion/1 -> BG/1
  Motion Based Background Estimator/2(Valid) -> Signal Conversion1/1
  Motion Based Background Estimator/1(BG) -> Signal Conversion/1
  In/1 -> Motion Based Background Estimator/1(In)

== system FlameAnalysis/Background Estimator/Decomposing Blue Movement/BG1/Temporal Median ==
  In : Inport
  Enable : EnablePort  PropagateVarSize=During execution
  Temporal Median : Subsystem  mask(Temporal Median){tw=52}
      mask prompts: tw "Enter the number of frames over which to compute the median:"
      mask help: Computes median values of a series of video frames.
      mask Display: disp('Temporal\nMedian')
  BG : Outport
  Valid : Outport  Port=2  InitialOutput=0
  wires:
  In/1 -> Temporal Median/1(In)
  Temporal Median/1(BG) -> BG/1
  Temporal Median/2(Valid) -> Valid/1

== system FlameAnalysis/Background Estimator/Decomposing Blue Movement/BG1/Temporal Median Estimator ==
  In : Inport
  Enable : EnablePort  PropagateVarSize=During execution
  Signal Conversion : SignalConversion  ConversionOutput=Contiguous copy
  Temporal Median Estimator : Subsystem  mask(Temporal Median Estimator){t0=2}
      mask prompts: t0 "Number of frames after which the median is valid:"
      mask help: This block estimates the median values of the video data over time. The accuracy of the estimate improves with each new video frame.
      mask Help:
      | The running median estimation algorithm updates the past median of time series data based upon the knowledge of the new data sample. The past median is incremented or decremented based on how the new sample compares to the old median by an amount determined by standard error of the estimate. A special correction is also applied when a local ramp is detected in the time series data attempting to push the estimate to follow the same ramp trend.
      | 
      | The estimated median is then constrained within Chebychev's bounds which are sqrt(3/5) of standard deviation either side of the mean of the data.
      mask Display: disp('Temporal\nMedian\nEstimator')
  BG : Outport
  Valid : Outport  Port=2  InitialOutput=0
  wires:
  Signal Conversion/1 -> BG/1
  Temporal Median Estimator/2(Valid) -> Valid/1
  Temporal Median Estimator/1(BG) -> Signal Conversion/1
  In/1 -> Temporal Median Estimator/1(In)

== system FlameAnalysis/Background Estimator/Decomposing Green Movement/BG1/Motion Based Background Estimator ==
  In : Inport
  Enable : EnablePort  PropagateVarSize=During execution
  Motion Based Background Estimator : Subsystem  mask(Motion Based Background Estimation){}
      mask help: The block uses the first few frames of the video stream to estimate the background image. It subtracts the background from each video frame to produce foreground images and only redraws the portion of the background that is revealed by the moving objects.
      mask Display: disp('Motion Based\nBackground\nEstimator')
  Signal Conversion : SignalConversion  ConversionOutput=Contiguous copy
  Signal Conversion1 : SignalConversion  ConversionOutput=Contiguous copy
  BG : Outport
  Valid : Outport  Port=2  InitialOutput=0
  wires:
  Signal Conversion1/1 -> Valid/1
  Signal Conversion/1 -> BG/1
  Motion Based Background Estimator/2(Valid) -> Signal Conversion1/1
  Motion Based Background Estimator/1(BG) -> Signal Conversion/1
  In/1 -> Motion Based Background Estimator/1(In)

== system FlameAnalysis/Background Estimator/Decomposing Green Movement/BG1/Temporal Median ==
  In : Inport
  Enable : EnablePort  PropagateVarSize=During execution
  Temporal Median : Subsystem  mask(Temporal Median){tw=52}
      mask prompts: tw "Enter the number of frames over which to compute the median:"
      mask help: Computes median values of a series of video frames.
      mask Display: disp('Temporal\nMedian')
  BG : Outport
  Valid : Outport  Port=2  InitialOutput=0
  wires:
  In/1 -> Temporal Median/1(In)
  Temporal Median/1(BG) -> BG/1
  Temporal Median/2(Valid) -> Valid/1

== system FlameAnalysis/Background Estimator/Decomposing Green Movement/BG1/Temporal Median Estimator ==
  In : Inport
  Enable : EnablePort  PropagateVarSize=During execution
  Signal Conversion : SignalConversion  ConversionOutput=Contiguous copy
  Temporal Median Estimator : Subsystem  mask(Temporal Median Estimator){t0=2}
      mask prompts: t0 "Number of frames after which the median is valid:"
      mask help: This block estimates the median values of the video data over time. The accuracy of the estimate improves with each new video frame.
      mask Help:
      | The running median estimation algorithm updates the past median of time series data based upon the knowledge of the new data sample. The past median is incremented or decremented based on how the new sample compares to the old median by an amount determined by standard error of the estimate. A special correction is also applied when a local ramp is detected in the time series data attempting to push the estimate to follow the same ramp trend.
      | 
      | The estimated median is then constrained within Chebychev's bounds which are sqrt(3/5) of standard deviation either side of the mean of the data.
      mask Display: disp('Temporal\nMedian\nEstimator')
  BG : Outport
  Valid : Outport  Port=2  InitialOutput=0
  wires:
  Signal Conversion/1 -> BG/1
  Temporal Median Estimator/2(Valid) -> Valid/1
  Temporal Median Estimator/1(BG) -> Signal Conversion/1
  In/1 -> Temporal Median Estimator/1(In)

== system FlameAnalysis/Background Estimator/Decomposing Red Movement/BG1/Motion Based Background Estimator ==
  In : Inport
  Enable : EnablePort  PropagateVarSize=During execution
  Motion Based Background Estimator : Subsystem  mask(Motion Based Background Estimation){}
      mask help: The block uses the first few frames of the video stream to estimate the background image. It subtracts the background from each video frame to produce foreground images and only redraws the portion of the background that is revealed by the moving objects.
      mask Display: disp('Motion Based\nBackground\nEstimator')
  Signal Conversion : SignalConversion  ConversionOutput=Contiguous copy
  Signal Conversion1 : SignalConversion  ConversionOutput=Contiguous copy
  BG : Outport
  Valid : Outport  Port=2  InitialOutput=0
  wires:
  Signal Conversion1/1 -> Valid/1
  Signal Conversion/1 -> BG/1
  Motion Based Background Estimator/2(Valid) -> Signal Conversion1/1
  Motion Based Background Estimator/1(BG) -> Signal Conversion/1
  In/1 -> Motion Based Background Estimator/1(In)

== system FlameAnalysis/Background Estimator/Decomposing Red Movement/BG1/Temporal Median ==
  In : Inport
  Enable : EnablePort  PropagateVarSize=During execution
  Temporal Median : Subsystem  mask(Temporal Median){tw=52}
      mask prompts: tw "Enter the number of frames over which to compute the median:"
      mask help: Computes median values of a series of video frames.
      mask Display: disp('Temporal\nMedian')
  BG : Outport
  Valid : Outport  Port=2  InitialOutput=0
  wires:
  In/1 -> Temporal Median/1(In)
  Temporal Median/1(BG) -> BG/1
  Temporal Median/2(Valid) -> Valid/1

== system FlameAnalysis/Background Estimator/Decomposing Red Movement/BG1/Temporal Median Estimator ==
  In : Inport
  Enable : EnablePort  PropagateVarSize=During execution
  Signal Conversion : SignalConversion  ConversionOutput=Contiguous copy
  Temporal Median Estimator : Subsystem  mask(Temporal Median Estimator){t0=2}
      mask prompts: t0 "Number of frames after which the median is valid:"
      mask help: This block estimates the median values of the video data over time. The accuracy of the estimate improves with each new video frame.
      mask Help:
      | The running median estimation algorithm updates the past median of time series data based upon the knowledge of the new data sample. The past median is incremented or decremented based on how the new sample compares to the old median by an amount determined by standard error of the estimate. A special correction is also applied when a local ramp is detected in the time series data attempting to push the estimate to follow the same ramp trend.
      | 
      | The estimated median is then constrained within Chebychev's bounds which are sqrt(3/5) of standard deviation either side of the mean of the data.
      mask Display: disp('Temporal\nMedian\nEstimator')
  BG : Outport
  Valid : Outport  Port=2  InitialOutput=0
  wires:
  Signal Conversion/1 -> BG/1
  Temporal Median Estimator/2(Valid) -> Valid/1
  Temporal Median Estimator/1(BG) -> Signal Conversion/1
  In/1 -> Temporal Median Estimator/1(In)

== system FlameAnalysis/Background Estimator/Decomposing Blue Movement/BG1/Motion Based Background Estimator/Motion Based Background Estimator ==
  In : Inport
  BG_running : Subsystem
  Logical Operator : Logic  Operator=NOT
  Unit Delay : UnitDelay  SampleTime=-1
  BG : Outport
  Valid : Outport  Port=2
  wires:
  Unit Delay/1 -> Logical Operator/1
  BG_running/1(BG) -> BG/1
  In/1 -> BG_running/1(In1)
  Logical Operator/1 -> BG_running/Enable
  BG_running/2(bgflag) -> Valid/1, Unit Delay/1

== system FlameAnalysis/Background Estimator/Decomposing Blue Movement/BG1/Temporal Median/Temporal Median ==
  In : Inport
  Background estimator : Subsystem  TreatAsAtomicUnit=on
  Logical Operator1 : Logic  Operator=NOT
  N-Sample Enale2 : Subsystem  mask(N Sample Enable){sample=tw}
      mask prompts: sample "Trigger Count, N"
      mask help: Active Level = Low(0)
  BG : Outport
  Valid : Outport  Port=2
  wires:
  In/1 -> Background estimator/1(Video In)
  Background estimator/1(Background) -> BG/1
  N-Sample Enale2/1(Enable) -> Background estimator/Enable, Logical Operator1/1
  Logical Operator1/1 -> Valid/1
